simulink model "FW_GCS_Sim"  (R2024b)
settings: Solver=ode4  StartTime=0.0  StopTime=inf  FixedStep=0.05  RelTol=1e-3
undefined symbols (not defined in the file): f
libraries: simulink x6, instrumentseriallib x4, instrumentlib x2, svdutilitieslib x1, aerolibanimutils x1, etargetslib x1, slrealtimeutilitieslib x1, xcpprotocollib x1
settings Model: Creator=tank2  LastModifiedBy=tank2
settings OptimizationCC: DefaultParameterBehavior=Inlined  EnhancedBackFolding=on  PassReuseOutputArgsAs=Individual arguments  ZeroExternalMemoryAtStartup=off  ZeroInternalMemoryAtStartup=off  OptimizeBlockOrder=speed  DifferentSizesBufferReuse=on  OptimizationCustomize=off  EfficientTunableParamExpr=on
settings DebuggingCC: ParameterTunabilityLossMsg=error
settings SFSimCC: MATLABDynamicMemAlloc=off
settings RTWCC: Description=Embedded Coder  SystemTargetFile=ert.tlc  TemplateMakefile=ert_default_tmf
settings CodeAppCC: ForceParamTrailComments=on  IgnoreCustomStorageClasses=off  OperatorAnnotations=on  SimulinkDataObjDesc=on  SFDataObjDesc=on  InsertBlockDesc=on
settings ERTTargetCC: TargetLangStandard=C99 (ISO)  GenerateSampleERTMain=on  ERTCustomFileTemplate=example_file_process.tlc

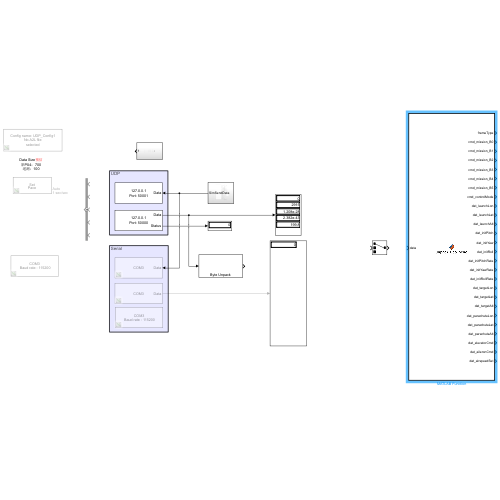
[thumbnail: Simulink's stored preview of the top-level diagram]
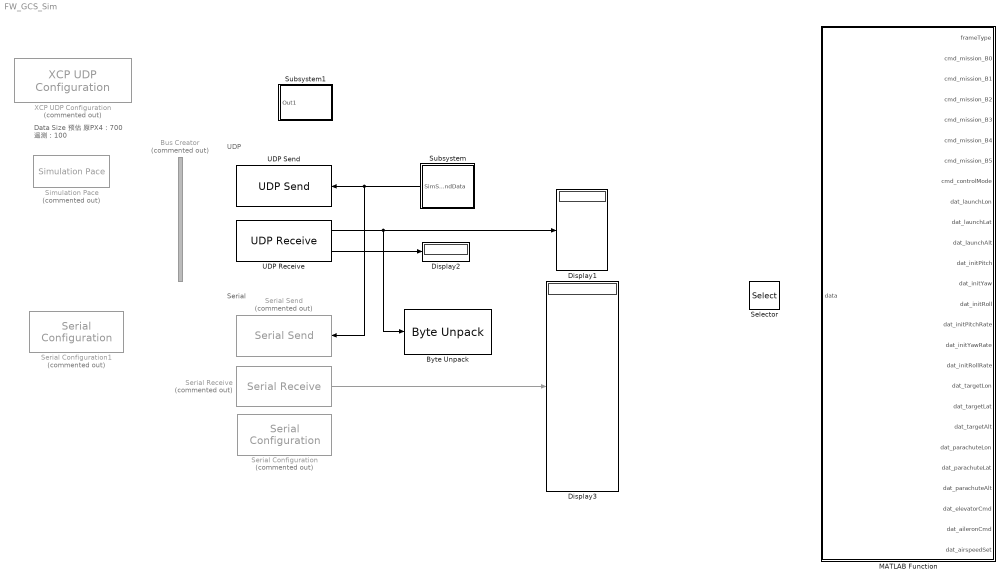
== system FW_GCS_Sim ==
  note: Serial
  note: UDP
  note: Data Size 预估
      | 原PX4：700
      | 遥测：100
  Bus Creator : BusCreator  Commented=on  Inputs=5  OutDataTypeStr=Bus: UdpRecvDataPacket_Bus
  Byte Unpack : svdutilitieslib/Byte Unpack  dimensions={[1]}  datatypes={'single'}  byteAlign=1  blockPlatform=tic2000
      settings: LibrarySourceBlock=c2000lib/Target Communication/Byte Unpack
  Display1 : Display
  Display2 : Display
  Display3 : Display
  MATLAB Function : MATLAB Function  TreatAsAtomicUnit=on
  Selector : Selector  InputPortWidth=3  IndexOptions=Starting index (dialog)  Indices=1  OutputSizes=1
  Serial Configuration : instrumentseriallib/Serial Configuration  Priority=-200000  Commented=on  PortSel=COM3  Port=COM3  ComPort=COM3  BaudRate=115200  DataBits=8  Parity=none  StopBits=1  ByteOrder=little-endian  FlowControl=none  Timeout=2  SimulateUsing=Interpreted execution  BlockInModel=on  aMode=1
      settings: LibrarySourceBlock=c2000lib/Host Communication/Serial Configuration
  Serial Configuration1 : instrumentseriallib/Serial Configuration  Priority=-200000  Commented=on  PortSel=COM3  Port=COM3  ComPort=COM3  BaudRate=115200  DataBits=8  Parity=none  StopBits=1  ByteOrder=little-endian  FlowControl=none  Timeout=10  SimulateUsing=Interpreted execution  BlockInModel=on  aMode=1
      settings: LibrarySourceBlock=c2000lib/Host Communication/Serial Configuration
  Serial Receive : instrumentseriallib/Serial Receive  Priority=1  Commented=on  PortSel=COM3  Port=COM3  ComPort=COM3  DataType=uint8  SaveDataType=uint8  ToggleHeader=on  Header=[0xFF, 0x00]  ToggleDataSize=on  DataSize=[800 1]  ToggleTerminator=off  Terminator=<none>  CustomTerminator=[]  InputFormat=Column major  EnableBlockingMode=on  ActionDataUnavailable=Output last received value  ActionWhenDataUnavailable=Output last received value  CustomValue=0  SampleTime=0.1  SimulateUsing=Interpreted execution  BlockInModel=on  aMode=1
      settings: LibrarySourceBlock=c2000lib/Host Communication/Serial Receive
  Serial Send : instrumentseriallib/Serial Send  Priority=1  Commented=on  PortSel=COM3  Port=COM3  ComPort=COM3  Header=[]  Terminator=<none>  CustomTerminator=[]  EnableBlockingMode=on  SimulateUsing=Interpreted execution  BlockInModel=on  aMode=1
      settings: LibrarySourceBlock=c2000lib/Host Communication/Serial Send
  Simulation Pace : aerolibanimutils/Simulation Pace  Commented=on  SimulationPace=1  SleepMode=Auto  OutputPaceError=off  SampleTime=-1
  Subsystem : Subsystem
  Subsystem1 : Subsystem
  UDP Receive : instrumentlib/UDP Receive  LocalAddress=127.0.0.1  LocalPort=50000  EnablePortSharing=off  Host=localhost  Port=50001  GetLatestData=off  DataSize=[1,5]  DataType=single  ASCIIFormatting=%f,  Terminator=LF  CustomTerminator=10  ByteOrder=little-endian  EnableBlockingMode=off  Timeout=30  SampleTime=0.25  SimulateUsing=Interpreted execution
  UDP Send : instrumentlib/UDP Send  Host=127.0.0.1  Port=50001  LocalAddress=127.0.0.1  LocalPort=50000  EnablePortSharing=off  OutputDatagramPacketSize=512  ByteOrder=big-endian  EnableBlockingMode=on  SimulateUsing=Interpreted execution
  XCP UDP Configuration : xcpprotocollib/UDP/XCP UDP Configuration  Priority=-100  Commented=on  SlaveName=UDP_Config1  SlaveID=1  EnableSecurity=off  ConnectMode=off  EnableStatus=off  SampleTime=-1  HeaderErrDet=on  CTRScheme=One counter for all CTOs and DTOs  LocalAddress=auto  LocalPort=auto  DAQTimeout=Inf
      settings: LibrarySourceBlock=xcprtlib/UDP/XCP UDP Configuration
  wires:
  UDP Receive/1 -> Display1/1, Byte Unpack/1
  UDP Receive/2 -> Display2/1
  Serial Receive/1 -> Display3/1
  Subsystem/1(SimSendData) -> UDP Send/1, Serial Send/1

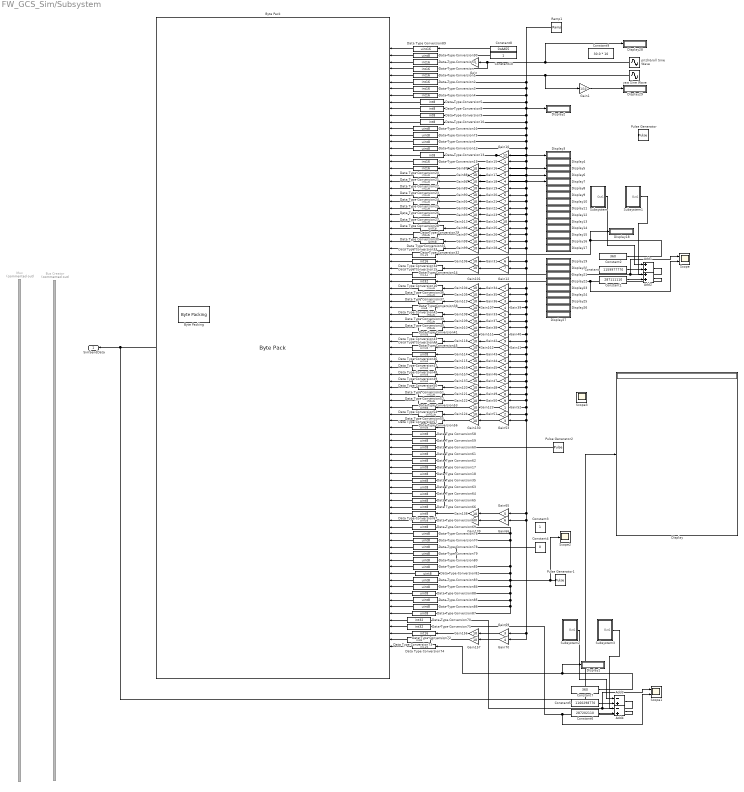
== system FW_GCS_Sim/Subsystem ==
  Add1 : Sum
  Add2 : Sum
  Add3 : Sum  Inputs=-+
  Add4 : Sum  Inputs=-+
  Bus Creator : BusCreator  Commented=on  Inputs=75
  Byte Pack : etargetslib/Byte Pack  datatypes="{    'uint16'    'uint8'    'int16'    'int16'    'int16'    'int16'    'int16'    'int16'    'int8'    'int8'    'int8'    'int8'    'uint8'    'uint8'    'uint8'    'uint8'    'int8'    'int16'    'int16'    'int16'    'int16'    'int16'    'int16'    'int16'    'int16'    'int16'    'int16'    'uint8'    'int16'    'uint8'    'uint8'    'int16'    'int16'    'uint8'    'int32'    'int32'    'int16'    'int16'    'int16'    'int8'    'int16'    'int16'    'int16'    'uint8'    'uint16'    'uint8'    'uint8'    'uint8'    'uint8'    'uint8'    'uint8'    'int16'    'int16'    'int16'    'uint8'    'uint16'    'uint16'    'uint8'    'uint8'    'uint8'    'uint8'    'uint8'    'uint8'    'uint8'    'uint8'    'uint8'    'uint8'    'uint8'    'uint8'    'uint8'    'uint8'    'uint8'    'uint8'    'uint8'    'uint8'    'uint8'    'uint8'    'uint8'    'uint8'    'uint8'    'uint8'    'uint8'    'uint8'    'uint8'    'uint8'    'uint8'    'int32'    'int32'    'int16'    'int8'    'int16'}"  byteAlign=1
  Byte Packing : slrealtimeutilitieslib/Byte Packing  MaskPackedDataType=uint8  MaskUnpackedDataTypes={'uint8'}  MaskAlignment=1
  Constant : Constant  Value=1159977770
  Constant1 : Constant  Value=287111110
  Constant10 : Constant
  Constant2 : Constant  Value=360
  Constant3 : Constant
  Constant4 : Constant  Value=0
  Constant5 : Constant  Value=1160298770
  Constant6 : Constant  Value=287202110
  Constant7 : Constant  Value=360
  Constant8 : Constant  Value=0xAA55
  Constant9 : Constant  Value=30.0 * 10
  Data Type Conversion{,1..4,7,19..28,30,33..34,36..41,51..53,72,74} (30 alike) : DataTypeConversion  OutDataTypeStr=int16  SaturateOnIntegerOverflow=off  RndMeth=Floor
  Data Type Conversion{5,8..10,13,42,73} (7 alike) : DataTypeConversion  OutDataTypeStr=int8  SaturateOnIntegerOverflow=off  RndMeth=Floor
  Data Type Conversion{6,11..12,14,17..18,29,31..32,35,43..44,46..50,54,57..69,75..88,90} (46 alike) : DataTypeConversion  OutDataTypeStr=uint8  SaturateOnIntegerOverflow=off  RndMeth=Floor
  Data Type Conversion{15..16,70..71} (4 alike) : DataTypeConversion  OutDataTypeStr=int32  SaturateOnIntegerOverflow=off  RndMeth=Floor
  Data Type Conversion{45,55..56,89} (4 alike) : DataTypeConversion  OutDataTypeStr=uint16  SaturateOnIntegerOverflow=off  RndMeth=Floor
  Display{,1..29} (30 alike) : Display
  Gain : Gain  Gain=-1
  Gain1 : Gain  Gain=1/10
  Gain10 : Gain  Gain=12
  Gain{24,87..94,96..99,101,104..124,130,137..139,156..157} (41 alike) : Gain  Gain=10
  Gain{12,21,38,48} (4 alike) : Gain  Gain=7
  Gain{15,25,34,41,52} (5 alike) : Gain
  Gain{16,26,35,43,51} (5 alike) : Gain  Gain=2
  Gain{17,27,36,44,53,69} (6 alike) : Gain  Gain=3
  Gain{18,28,39,45,70} (5 alike) : Gain  Gain=4
  Gain{19,33,46,65} (4 alike) : Gain  Gain=5
  Gain{20,31,37,47,66} (5 alike) : Gain  Gain=6
  Gain22 : Gain  Gain=8
  Gain23 : Gain  Gain=9
  Gain40 : Gain  Gain=8
  Gain42 : Gain  Gain=9
  Gain49 : Gain  Gain=8
  Gain50 : Gain  Gain=9
  Mux : Mux  Commented=on  Inputs=75
  Pulse Generator : DiscretePulseGenerator  PulseType=Time based  Period=3  PulseWidth=5
  Pulse Generator1 : DiscretePulseGenerator  PulseType=Time based  Period=300  PulseWidth=5
  Pulse Generator2 : DiscretePulseGenerator  PulseType=Time based  Period=5  PulseWidth=50
  Ramp1 : simulink/Sources/Ramp  slope=0.1  start=0  InitialOutput=1
  Scope : Scope  NumInputPorts=2
  Scope1 : Scope  NumInputPorts=2
  Scope2 : Scope
  Scope3 : Scope
  Subsystem : Subsystem
  Subsystem1 : Subsystem
  Subsystem2 : Subsystem
  Subsystem3 : Subsystem
  pitch&roll Sine Wave : Sin  Amplitude=89*10  Frequency=0.01047/2  SampleTime=0
  yaw Sine Wave : Sin  Amplitude=180*10  Bias=180*10  Frequency=0.01047  SampleTime=0
  SimSendData : Outport
  wires:
  Gain16/1 -> Gain87/1
  Gain17/1 -> Gain88/1
  Gain18/1 -> Gain94/1
  Gain19/1 -> Gain89/1
  Gain20/1 -> Gain90/1
  Gain23/1 -> Gain93/1
  Gain22/1 -> Gain92/1
  Gain21/1 -> Gain91/1
  Gain24/1 -> Gain113/1
  Gain26/1 -> Gain97/1
  Gain25/1 -> Gain96/1
  Gain27/1 -> Gain98/1
  Gain28/1 -> Gain99/1
  Gain31/1 -> Gain106/1
  Gain12/1 -> Gain101/1
  Gain34/1 -> Gain104/1
  Gain35/1 -> Gain105/1
  Gain36/1 -> Gain119/1
  Gain37/1 -> Gain109/1
  Gain33/1 -> Gain108/1
  Gain38/1 -> Gain110/1
  Gain39/1 -> Gain107/1
  Gain40/1 -> Gain111/1
  Gain41/1 -> Gain112/1
  Gain42/1 -> Gain118/1
  Gain43/1 -> Gain114/1
  Gain45/1 -> Gain116/1
  Gain44/1 -> Gain115/1
  Gain46/1 -> Gain117/1
  Gain47/1 -> Gain137/1
  Gain48/1 -> Gain120/1
  Gain50/1 -> Gain122/1
  Gain49/1 -> Gain121/1
  Gain52/1 -> Gain123/1
  Gain51/1 -> Gain124/1
  Gain53/1 -> Gain130/1
  Gain66/1 -> Gain139/1
  Gain65/1 -> Gain138/1
  Gain69/1 -> Gain156/1
  Gain70/1 -> Gain157/1
  Byte Pack/1 -> Display/1, SimSendData/1
  Gain92/1 -> Data Type Conversion26/1
  Gain91/1 -> Data Type Conversion25/1
  Gain96/1 -> Data Type Conversion29/1
  Gain97/1 -> Data Type Conversion30/1
  Gain99/1 -> Data Type Conversion32/1
  Gain98/1 -> Data Type Conversion31/1
  Gain94/1 -> Display7/1, Data Type Conversion22/1
  Gain93/1 -> Data Type Conversion27/1
  Gain90/1 -> Data Type Conversion24/1
  Gain101/1 -> Data Type Conversion14/1
  Gain106/1 -> Data Type Conversion34/1
  Gain105/1 -> Data Type Conversion37/1
  Gain107/1 -> Data Type Conversion42/1
  Gain104/1 -> Data Type Conversion36/1
  Gain116/1 -> Data Type Conversion48/1
  Gain113/1 -> Data Type Conversion28/1
  Gain108/1 -> Data Type Conversion39/1
  Gain110/1 -> Data Type Conversion41/1
  Gain111/1 -> Data Type Conversion43/1
  Gain112/1 -> Data Type Conversion44/1
  Gain114/1 -> Data Type Conversion46/1
  Gain109/1 -> Data Type Conversion40/1
  Gain115/1 -> Data Type Conversion47/1
  Gain119/1 -> Data Type Conversion38/1
  Gain120/1 -> Data Type Conversion51/1
  Gain117/1 -> Data Type Conversion49/1
  Gain121/1 -> Data Type Conversion52/1
  Gain118/1 -> Data Type Conversion45/1
  Gain122/1 -> Data Type Conversion53/1
  Gain123/1 -> Data Type Conversion54/1
  Gain124/1 -> Data Type Conversion55/1
  Gain130/1 -> Data Type Conversion56/1
  Gain139/1 -> Data Type Conversion68/1
  Gain138/1 -> Data Type Conversion67/1
  Gain137/1 -> Data Type Conversion50/1
  Gain157/1 -> Data Type Conversion73/1
  Pulse Generator1/1 -> Data Type Conversion83/1, Data Type Conversion82/1, Data Type Conversion81/1, Data Type Conversion76/1, Data Type Conversion69/1, Data Type Conversion77/1, Data Type Conversion84/1, Data Type Conversion88/1, Data Type Conversion85/1, Data Type Conversion86/1, Data Type Conversion87/1, Scope2/1
  Gain156/1 -> Data Type Conversion72/1
  Gain87/1 -> Data Type Conversion20/1, Display5/1
  Gain89/1 -> Data Type Conversion23/1
  Gain88/1 -> Data Type Conversion21/1, Display6/1
  Gain10/1 -> Data Type Conversion13/1, Display3/1
  Gain15/1 -> Data Type Conversion19/1
  Ramp1/1 -> Display2/1, Data Type Conversion8/1, Data Type Conversion9/1, Data Type Conversion10/1, Data Type Conversion75/1, Data Type Conversion6/1, Gain10/1, Gain39/1, Gain43/1, Gain45/1, Gain53/1, Gain65/1, Gain70/1, Gain69/1, Gain66/1, Gain51/1, Gain52/1, Gain50/1, Gain49/1, Gain48/1, Gain47/1, Gain46/1, Gain44/1, Gain41/1, Gain42/1, Gain40/1, Gain38/1, Gain37/1, Gain33/1, Gain36/1, Gain35/1, Gain34/1, Gain12/1, Gain31/1, Gain28/1, Gain27/1, Gain26/1, Gain25/1, Gain24/1, Gain23/1, Gain22/1, Gain21/1, Gain20/1, Gain19/1, Gain18/1, Gain17/1, Gain16/1, Gain15/1, Data Type Conversion12/1, Data Type Conversion11/1, Data Type Conversion5/1, Data Type Conversion4/1, Data Type Conversion3/1, Data Type Conversion2/1
  Constant1/1 -> Add2/2
  Constant/1 -> Add1/2
  Constant2/1 -> Data Type Conversion33/1, Display18/1
  Add1/1 -> Data Type Conversion15/1, Scope/1
  Add2/1 -> Scope/2, Data Type Conversion16/1
  Subsystem/1(Out1) -> Add1/1
  Subsystem1/1(Out1) -> Add2/1
  Constant4/1 -> Data Type Conversion80/1, Data Type Conversion79/1, Data Type Conversion78/1
  Subsystem3/1(Out1) -> Add4/1
  Add3/1 -> Data Type Conversion70/1, Scope1/1
  Constant6/1 -> Add4/2
  Add4/1 -> Data Type Conversion71/1, Scope1/2
  Constant7/1 -> Display1/1, Data Type Conversion74/1
  Constant5/1 -> Add3/2
  Subsystem2/1(Out1) -> Add3/1
  Constant8/1 -> Data Type Conversion89/1
  Pulse Generator2/1 -> Data Type Conversion62/1, Data Type Conversion17/1, Data Type Conversion18/1, Data Type Conversion35/1, Data Type Conversion63/1, Data Type Conversion64/1, Data Type Conversion65/1, Data Type Conversion66/1, Data Type Conversion61/1, Data Type Conversion58/1, Data Type Conversion57/1, Data Type Conversion59/1, Data Type Conversion60/1
  pitch&roll Sine Wave/1 -> Display28/1, Data Type Conversion/1, Gain/1
  yaw Sine Wave/1 -> Gain1/1, Data Type Conversion1/1
  Gain/1 -> Data Type Conversion7/1
  Gain1/1 -> Display29/1
  Data Type Conversion70/1 -> Byte Pack/87
  Data Type Conversion71/1 -> Byte Pack/88
  Data Type Conversion73/1 -> Byte Pack/90
  Data Type Conversion89/1 -> Byte Pack/1
  Constant10/1 -> Data Type Conversion90/1
  Data Type Conversion90/1 -> Byte Pack/2
  Data Type Conversion7/1 -> Byte Pack/3
  Data Type Conversion/1 -> Byte Pack/4
  Data Type Conversion1/1 -> Byte Pack/5
  Data Type Conversion2/1 -> Byte Pack/6
  Data Type Conversion3/1 -> Byte Pack/7
  Data Type Conversion4/1 -> Byte Pack/8
  Data Type Conversion5/1 -> Byte Pack/9
  Data Type Conversion8/1 -> Byte Pack/10
  Data Type Conversion9/1 -> Byte Pack/11
  Data Type Conversion10/1 -> Byte Pack/12
  Data Type Conversion11/1 -> Byte Pack/13
  Data Type Conversion75/1 -> Byte Pack/14
  Data Type Conversion6/1 -> Byte Pack/15
  Data Type Conversion12/1 -> Byte Pack/16
  Data Type Conversion13/1 -> Byte Pack/17
  Data Type Conversion19/1 -> Byte Pack/18
  Data Type Conversion20/1 -> Byte Pack/19
  Data Type Conversion21/1 -> Byte Pack/20
  Data Type Conversion22/1 -> Byte Pack/21
  Data Type Conversion23/1 -> Byte Pack/22
  Data Type Conversion24/1 -> Byte Pack/23
  Data Type Conversion25/1 -> Byte Pack/24
  Data Type Conversion26/1 -> Byte Pack/25
  Data Type Conversion27/1 -> Byte Pack/26
  Data Type Conversion28/1 -> Byte Pack/27
  Data Type Conversion29/1 -> Byte Pack/28
  Data Type Conversion30/1 -> Byte Pack/29
  Data Type Conversion31/1 -> Byte Pack/30
  Data Type Conversion32/1 -> Byte Pack/31
  Data Type Conversion33/1 -> Byte Pack/32
  Data Type Conversion34/1 -> Byte Pack/33
  Data Type Conversion14/1 -> Byte Pack/34
  Data Type Conversion15/1 -> Byte Pack/35
  Data Type Conversion16/1 -> Byte Pack/36
  Data Type Conversion36/1 -> Byte Pack/37
  Data Type Conversion37/1 -> Byte Pack/38
  Data Type Conversion38/1 -> Byte Pack/39
  Data Type Conversion42/1 -> Byte Pack/40
  Data Type Conversion39/1 -> Byte Pack/41
  Data Type Conversion40/1 -> Byte Pack/42
  Data Type Conversion41/1 -> Byte Pack/43
  Data Type Conversion43/1 -> Byte Pack/44
  Data Type Conversion45/1 -> Byte Pack/45
  Data Type Conversion44/1 -> Byte Pack/46
  Data Type Conversion46/1 -> Byte Pack/47
  Data Type Conversion47/1 -> Byte Pack/48
  Data Type Conversion48/1 -> Byte Pack/49
  Data Type Conversion49/1 -> Byte Pack/50
  Data Type Conversion50/1 -> Byte Pack/51
  Data Type Conversion51/1 -> Byte Pack/52
  Data Type Conversion52/1 -> Byte Pack/53
  Data Type Conversion53/1 -> Byte Pack/54
  Data Type Conversion54/1 -> Byte Pack/55
  Data Type Conversion55/1 -> Byte Pack/56
  Data Type Conversion56/1 -> Byte Pack/57
  Data Type Conversion57/1 -> Byte Pack/58
  Data Type Conversion58/1 -> Byte Pack/59
  Data Type Conversion59/1 -> Byte Pack/60
  Data Type Conversion60/1 -> Byte Pack/61
  Data Type Conversion61/1 -> Byte Pack/62
  Data Type Conversion62/1 -> Byte Pack/63
  Data Type Conversion17/1 -> Byte Pack/64
  Data Type Conversion18/1 -> Byte Pack/65
  Data Type Conversion35/1 -> Byte Pack/66
  Data Type Conversion63/1 -> Byte Pack/67
  Data Type Conversion64/1 -> Byte Pack/68
  Data Type Conversion65/1 -> Byte Pack/69
  Data Type Conversion66/1 -> Byte Pack/70
  Data Type Conversion69/1 -> Byte Pack/73
  Data Type Conversion68/1 -> Byte Pack/72
  Data Type Conversion67/1 -> Byte Pack/71
  Data Type Conversion76/1 -> Byte Pack/74
  Data Type Conversion77/1 -> Byte Pack/75
  Data Type Conversion78/1 -> Byte Pack/76
  Data Type Conversion79/1 -> Byte Pack/77
  Data Type Conversion80/1 -> Byte Pack/78
  Data Type Conversion81/1 -> Byte Pack/79
  Data Type Conversion82/1 -> Byte Pack/80
  Data Type Conversion83/1 -> Byte Pack/81
  Data Type Conversion84/1 -> Byte Pack/82
  Data Type Conversion88/1 -> Byte Pack/83
  Data Type Conversion85/1 -> Byte Pack/84
  Data Type Conversion86/1 -> Byte Pack/85
  Data Type Conversion87/1 -> Byte Pack/86
  Data Type Conversion72/1 -> Byte Pack/89
  Data Type Conversion74/1 -> Byte Pack/91

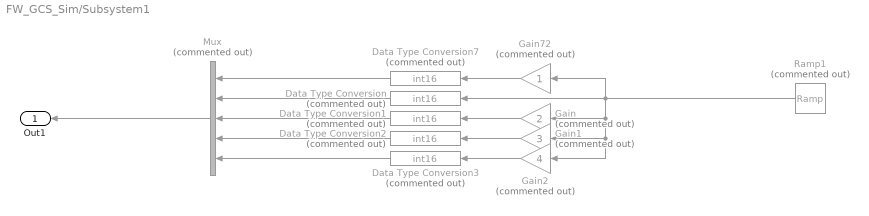
== system FW_GCS_Sim/Subsystem1 ==
  Data Type Conversion{,1..3,7} (5 alike) : DataTypeConversion  Commented=on  OutDataTypeStr=int16  SaturateOnIntegerOverflow=off  RndMeth=Floor
  Gain : Gain  Commented=on  Gain=2
  Gain1 : Gain  Commented=on  Gain=3
  Gain2 : Gain  Commented=on  Gain=4
  Gain72 : Gain  Commented=on
  Mux : Mux  Commented=on  Inputs=5
  Ramp1 : simulink/Sources/Ramp  Commented=on  slope=1  start=0  InitialOutput=0
  Out1 : Outport
  wires:
  Data Type Conversion2/1 -> Mux/4
  Ramp1/1 -> Gain72/1, Gain2/1, Gain1/1, Gain/1, Data Type Conversion/1
  Data Type Conversion1/1 -> Mux/3
  Data Type Conversion7/1 -> Mux/1
  Gain72/1 -> Data Type Conversion7/1
  Data Type Conversion/1 -> Mux/2
  Data Type Conversion3/1 -> Mux/5
  Gain1/1 -> Data Type Conversion2/1
  Gain/1 -> Data Type Conversion1/1
  Gain2/1 -> Data Type Conversion3/1
  Mux/1 -> Out1/1

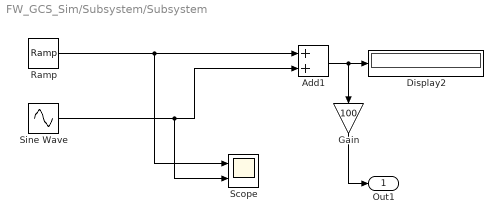
== system FW_GCS_Sim/Subsystem/Subsystem ==
  Add1 : Sum
  Display2 : Display
  Gain : Gain  Gain=100
  Ramp : simulink/Sources/Ramp  slope=1  start=0  InitialOutput=0
  Scope : Scope  NumInputPorts=2
  Sine Wave : Sin  Amplitude=500  Frequency=0.0001  SampleTime=0
  Out1 : Outport
  wires:
  Ramp/1 -> Scope/1, Add1/1
  Sine Wave/1 -> Scope/2, Add1/2
  Add1/1 -> Display2/1, Gain/1
  Gain/1 -> Out1/1

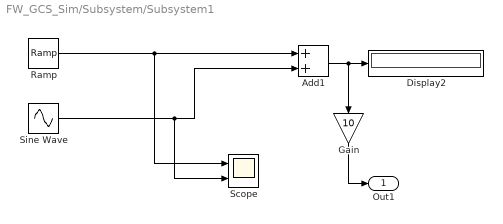
== system FW_GCS_Sim/Subsystem/Subsystem1 ==
  Add1 : Sum
  Display2 : Display
  Gain : Gain  Gain=10
  Ramp : simulink/Sources/Ramp  slope=-1  start=0  InitialOutput=0
  Scope : Scope  NumInputPorts=2
  Sine Wave : Sin  Amplitude=700  Frequency=0.01  SampleTime=0
  Out1 : Outport
  wires:
  Ramp/1 -> Scope/1, Add1/1
  Sine Wave/1 -> Scope/2, Add1/2
  Add1/1 -> Display2/1, Gain/1
  Gain/1 -> Out1/1

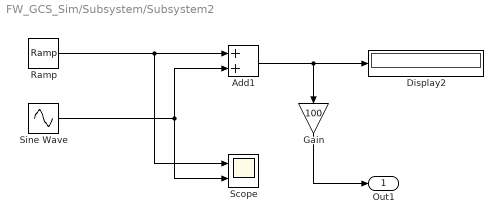
== system FW_GCS_Sim/Subsystem/Subsystem2 ==
  Add1 : Sum
  Display2 : Display
  Gain : Gain  Gain=100
  Ramp : simulink/Sources/Ramp  slope=1  start=0  InitialOutput=0
  Scope : Scope  NumInputPorts=2
  Sine Wave : Sin  Amplitude=200  Frequency=0.0001  SampleTime=0
  Out1 : Outport
  wires:
  Ramp/1 -> Scope/1, Add1/1
  Sine Wave/1 -> Scope/2, Add1/2
  Add1/1 -> Display2/1, Gain/1
  Gain/1 -> Out1/1

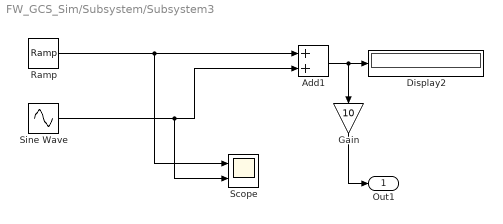
== system FW_GCS_Sim/Subsystem/Subsystem3 ==
  Add1 : Sum
  Display2 : Display
  Gain : Gain  Gain=10
  Ramp : simulink/Sources/Ramp  slope=-1  start=0  InitialOutput=0
  Scope : Scope  NumInputPorts=2
  Sine Wave : Sin  Amplitude=300  Frequency=0.01  SampleTime=0
  Out1 : Outport
  wires:
  Ramp/1 -> Scope/1, Add1/1
  Sine Wave/1 -> Scope/2, Add1/2
  Add1/1 -> Display2/1, Gain/1
  Gain/1 -> Out1/1

== matlab function FW_GCS_Sim/MATLAB Function ==
  data: data input; frameType output; cmd_mission_B0 output; cmd_mission_B1 output; cmd_mission_B2 output; cmd_mission_B3 output; cmd_mission_B4 output; cmd_mission_B5 output; cmd_controlMode output; dat_launchLon output; dat_launchLat output; dat_launchAlt output; dat_initPitch output; dat_initYaw output; dat_initRoll output; dat_initPitchRate output; dat_initYawRate output; dat_initRollRate output; dat_targetLon output; dat_targetLat output; dat_targetAlt output; dat_parachuteLon output; dat_parachuteLat output; dat_parachuteAlt output; dat_elevatorCmd output; dat_aileronCmd output; dat_airspeedSet output
function [frameType, cmd_mission_B0, cmd_mission_B1, cmd_mission_B2, cmd_mission_B3, cmd_mission_B4, cmd_mission_B5, cmd_controlMode, dat_launchLon, dat_launchLat, dat_launchAlt, dat_initPitch, dat_initYaw, dat_initRoll, dat_initPitchRate, dat_initYawRate, dat_initRollRate, dat_targetLon, dat_targetLat, dat_targetAlt, dat_parachuteLon, dat_parachuteLat, dat_parachuteAlt, dat_elevatorCmd, dat_aileronCmd, dat_airspeedSet] = unpack_udp_send(data)
